simulink model "lab4_4"  (R2017b)
settings: Solver=VariableStepAuto  StartTime=0.0  StopTime=4  RelTol=1e-3
settings Model: Creator=yoel_  LastModifiedBy=yoel_

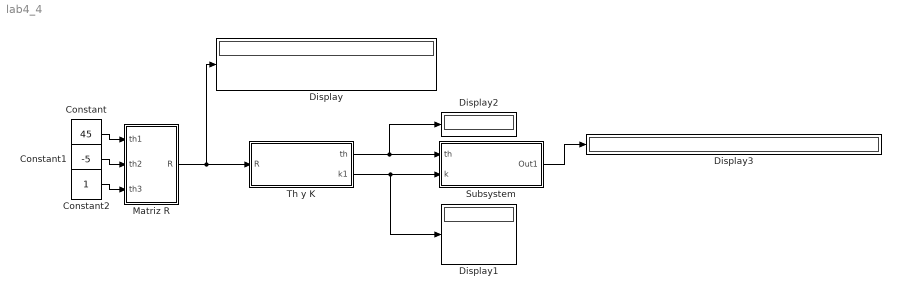
== system lab4_4 ==
  Constant : Constant  Value=45
  Constant1 : Constant  Value=-5
  Constant2 : Constant
  Display{,1..3} (4 alike) : Display
  Matriz R : Subsystem
  Subsystem : Subsystem
  Th y K : Subsystem
  wires:
  Constant/1 -> Matriz R/1(th1)
  Constant1/1 -> Matriz R/2(th2)
  Constant2/1 -> Matriz R/3(th3)
  Matriz R/1(R) -> Th y K/1("R "), Display/1
  Th y K/2(k1) -> Subsystem/2("k "), Display1/1
  Th y K/1("th ") -> Subsystem/1("th "), Display2/1
  Subsystem/1(Out1) -> Display3/1

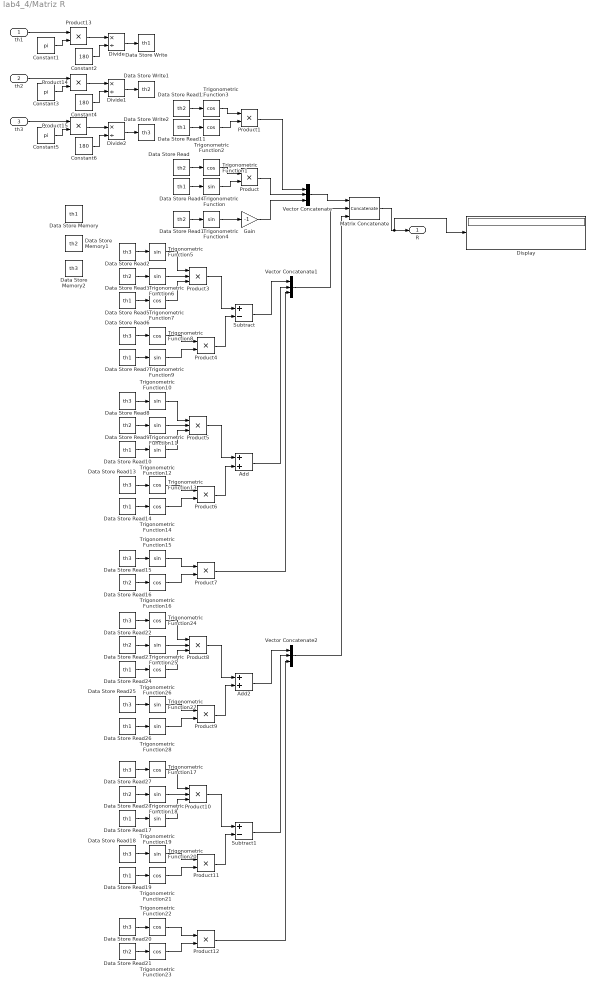
== system lab4_4/Matriz R ==
  th1 : Inport
  th2 : Inport  Port=2
  th3 : Inport  Port=3
  Add : Sum
  Add2 : Sum
  Constant1 : Constant  Value=pi
  Constant2 : Constant  Value=180
  Constant3 : Constant  Value=pi
  Constant4 : Constant  Value=180
  Constant5 : Constant  Value=pi
  Constant6 : Constant  Value=180
  Data Store Memory : DataStoreMemory  DataStoreName=th1  ReadBeforeWriteMsg=warning  WriteAfterWriteMsg=warning  WriteAfterReadMsg=warning  ShowAdditionalParam=off
  Data Store Memory1 : DataStoreMemory  DataStoreName=th2  ReadBeforeWriteMsg=warning  WriteAfterWriteMsg=warning  WriteAfterReadMsg=warning  ShowAdditionalParam=off
  Data Store Memory2 : DataStoreMemory  DataStoreName=th3  ReadBeforeWriteMsg=warning  WriteAfterWriteMsg=warning  WriteAfterReadMsg=warning  ShowAdditionalParam=off
  Data Store Read{,1,3,9,12,16,21,23,28} (9 alike) : DataStoreRead  DataStoreName=th2
  Data Store Read{4..5,7,10..11,14,17,19,24,26} (10 alike) : DataStoreRead  DataStoreName=th1
  Data Store Read{2,6,8,13,15,18,20,22,25,27} (10 alike) : DataStoreRead  DataStoreName=th3
  Data Store Write : DataStoreWrite  DataStoreName=th1
  Data Store Write1 : DataStoreWrite  DataStoreName=th2
  Data Store Write2 : DataStoreWrite  DataStoreName=th3
  Display : Display
  Divide : Product  Inputs=*/
  Divide1 : Product  Inputs=*/
  Divide2 : Product  Inputs=*/
  Gain : Gain  Gain=-1
  Matrix Concatenate : Concatenate  NumInputs=3  ConcatenateDimension=3
  Product{,1,4,6..7,9,11..15} (11 alike) : Product
  Product{3,5,8,10} (4 alike) : Product  Inputs=3
  Subtract : Sum  Inputs=+-
  Subtract1 : Sum  Inputs=+-
  Trigonometric Function{,4..6,9..12,15,18..20,25,27..28} (15 alike) : Trigonometry
  Trigonometric Function{1..3,7..8,13..14,16..17,21..24,26} (14 alike) : Trigonometry  Operator=cos
  Vector Concatenate : Concatenate  NumInputs=3
  Vector Concatenate1 : Concatenate  NumInputs=3
  Vector Concatenate2 : Concatenate  NumInputs=3
  R : Outport
  wires:
  Trigonometric Function3/1 -> Product1/1
  Trigonometric Function/1 -> Product/2
  Trigonometric Function2/1 -> Product1/2
  Trigonometric Function1/1 -> Product/1
  Trigonometric Function4/1 -> Gain/1
  Data Store Read12/1 -> Trigonometric Function3/1
  Data Store Read11/1 -> Trigonometric Function2/1
  Data Store Read/1 -> Trigonometric Function1/1
  Data Store Read4/1 -> Trigonometric Function/1
  Data Store Read1/1 -> Trigonometric Function4/1
  Product1/1 -> Vector Concatenate/1
  Product/1 -> Vector Concatenate/2
  Gain/1 -> Vector Concatenate/3
  Vector Concatenate/1 -> Matrix Concatenate/1
  Vector Concatenate1/1 -> Matrix Concatenate/2
  Matrix Concatenate/1 -> Display/1, R/1
  Data Store Read2/1 -> Trigonometric Function5/1
  Data Store Read3/1 -> Trigonometric Function6/1
  Data Store Read5/1 -> Trigonometric Function7/1
  Trigonometric Function5/1 -> Product3/1
  Trigonometric Function6/1 -> Product3/2
  Trigonometric Function7/1 -> Product3/3
  Product3/1 -> Subtract/1
  Data Store Read6/1 -> Trigonometric Function8/1
  Data Store Read7/1 -> Trigonometric Function9/1
  Trigonometric Function8/1 -> Product4/1
  Trigonometric Function9/1 -> Product4/2
  Product4/1 -> Subtract/2
  Subtract/1 -> Vector Concatenate1/1
  Product6/1 -> Add/2
  Trigonometric Function11/1 -> Product5/2
  Data Store Read9/1 -> Trigonometric Function11/1
  Trigonometric Function14/1 -> Product6/2
  Trigonometric Function12/1 -> Product5/3
  Data Store Read14/1 -> Trigonometric Function14/1
  Data Store Read10/1 -> Trigonometric Function12/1
  Trigonometric Function13/1 -> Product6/1
  Product5/1 -> Add/1
  Data Store Read8/1 -> Trigonometric Function10/1
  Trigonometric Function10/1 -> Product5/1
  Data Store Read13/1 -> Trigonometric Function13/1
  Add/1 -> Vector Concatenate1/2
  Data Store Read15/1 -> Trigonometric Function15/1
  Data Store Read16/1 -> Trigonometric Function16/1
  Trigonometric Function15/1 -> Product7/1
  Trigonometric Function16/1 -> Product7/2
  Product7/1 -> Vector Concatenate1/3
  Product12/1 -> Vector Concatenate2/3
  Trigonometric Function23/1 -> Product12/2
  Trigonometric Function22/1 -> Product12/1
  Data Store Read21/1 -> Trigonometric Function23/1
  Data Store Read20/1 -> Trigonometric Function22/1
  Subtract1/1 -> Vector Concatenate2/2
  Data Store Read18/1 -> Trigonometric Function20/1
  Trigonometric Function17/1 -> Product10/1
  Data Store Read27/1 -> Trigonometric Function17/1
  Product10/1 -> Subtract1/1
  Trigonometric Function20/1 -> Product11/1
  Data Store Read17/1 -> Trigonometric Function19/1
  Data Store Read19/1 -> Trigonometric Function21/1
  Trigonometric Function19/1 -> Product10/3
  Trigonometric Function21/1 -> Product11/2
  Data Store Read28/1 -> Trigonometric Function18/1
  Trigonometric Function18/1 -> Product10/2
  Product11/1 -> Subtract1/2
  Add2/1 -> Vector Concatenate2/1
  Product9/1 -> Add2/2
  Trigonometric Function28/1 -> Product9/2
  Trigonometric Function27/1 -> Product9/1
  Data Store Read26/1 -> Trigonometric Function28/1
  Data Store Read25/1 -> Trigonometric Function27/1
  Product8/1 -> Add2/1
  Trigonometric Function26/1 -> Product8/3
  Trigonometric Function25/1 -> Product8/2
  Trigonometric Function24/1 -> Product8/1
  Data Store Read24/1 -> Trigonometric Function26/1
  Data Store Read23/1 -> Trigonometric Function25/1
  Data Store Read22/1 -> Trigonometric Function24/1
  Vector Concatenate2/1 -> Matrix Concatenate/3
  th1/1 -> Product13/1
  Constant1/1 -> Product13/2
  Product13/1 -> Divide/1
  Constant2/1 -> Divide/2
  Divide/1 -> Data Store Write/1
  Divide1/1 -> Data Store Write1/1
  Constant4/1 -> Divide1/2
  Product14/1 -> Divide1/1
  Constant3/1 -> Product14/2
  th2/1 -> Product14/1
  th3/1 -> Product15/1
  Constant5/1 -> Product15/2
  Product15/1 -> Divide2/1
  Constant6/1 -> Divide2/2
  Divide2/1 -> Data Store Write2/1

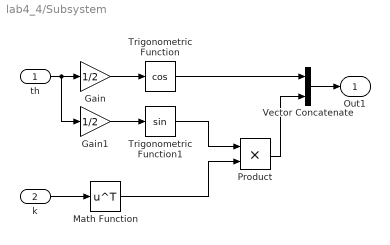
== system lab4_4/Subsystem ==
  "th " : Inport
  "k " : Inport  Port=2
  Gain : Gain  Gain=1/2
  Gain1 : Gain  Gain=1/2
  Math Function : Math  Operator=transpose  SaturateOnIntegerOverflow=on
  Product : Product
  Trigonometric Function : Trigonometry  Operator=cos
  Trigonometric Function1 : Trigonometry
  Vector Concatenate : Concatenate
  Out1 : Outport
  wires:
  "th "/1 -> Gain1/1, Gain/1
  Gain/1 -> Trigonometric Function/1
  Gain1/1 -> Trigonometric Function1/1
  "k "/1 -> Math Function/1
  Trigonometric Function1/1 -> Product/1
  Math Function/1 -> Product/2
  Product/1 -> Vector Concatenate/2
  Trigonometric Function/1 -> Vector Concatenate/1
  Vector Concatenate/1 -> Out1/1

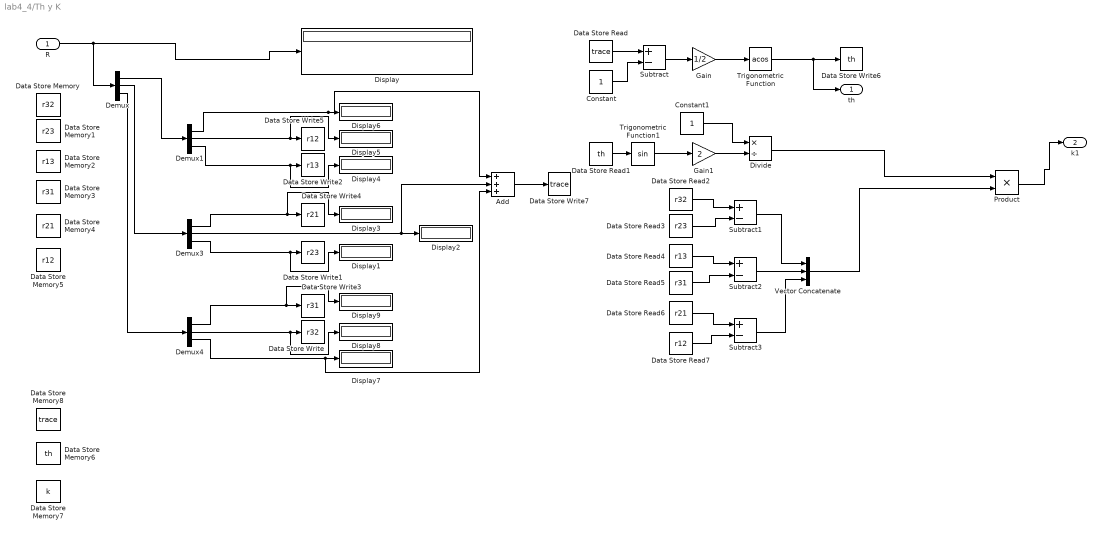
== system lab4_4/Th y K ==
  "R " : Inport
  Add : Sum  Inputs=3
  Constant : Constant
  Constant1 : Constant
  Data Store Memory : DataStoreMemory  DataStoreName=r32  ReadBeforeWriteMsg=warning  WriteAfterWriteMsg=warning  WriteAfterReadMsg=warning  ShowAdditionalParam=off
  Data Store Memory1 : DataStoreMemory  DataStoreName=r23  ReadBeforeWriteMsg=warning  WriteAfterWriteMsg=warning  WriteAfterReadMsg=warning  ShowAdditionalParam=off
  Data Store Memory2 : DataStoreMemory  DataStoreName=r13  ReadBeforeWriteMsg=warning  WriteAfterWriteMsg=warning  WriteAfterReadMsg=warning  ShowAdditionalParam=off
  Data Store Memory3 : DataStoreMemory  DataStoreName=r31  ReadBeforeWriteMsg=warning  WriteAfterWriteMsg=warning  WriteAfterReadMsg=warning  ShowAdditionalParam=off
  Data Store Memory4 : DataStoreMemory  DataStoreName=r21  ReadBeforeWriteMsg=warning  WriteAfterWriteMsg=warning  WriteAfterReadMsg=warning  ShowAdditionalParam=off
  Data Store Memory5 : DataStoreMemory  DataStoreName=r12  ReadBeforeWriteMsg=warning  WriteAfterWriteMsg=warning  WriteAfterReadMsg=warning  ShowAdditionalParam=off
  Data Store Memory6 : DataStoreMemory  DataStoreName=th  ReadBeforeWriteMsg=warning  WriteAfterWriteMsg=warning  WriteAfterReadMsg=warning  ShowAdditionalParam=off
  Data Store Memory7 : DataStoreMemory  DataStoreName=k  ReadBeforeWriteMsg=warning  WriteAfterWriteMsg=warning  WriteAfterReadMsg=warning  ShowAdditionalParam=off
  Data Store Memory8 : DataStoreMemory  DataStoreName=trace  ReadBeforeWriteMsg=warning  WriteAfterWriteMsg=warning  WriteAfterReadMsg=warning  ShowAdditionalParam=off
  Data Store Read : DataStoreRead  DataStoreName=trace
  Data Store Read1 : DataStoreRead  DataStoreName=th
  Data Store Read2 : DataStoreRead  DataStoreName=r32
  Data Store Read3 : DataStoreRead  DataStoreName=r23
  Data Store Read4 : DataStoreRead  DataStoreName=r13
  Data Store Read5 : DataStoreRead  DataStoreName=r31
  Data Store Read6 : DataStoreRead  DataStoreName=r21
  Data Store Read7 : DataStoreRead  DataStoreName=r12
  Data Store Write : DataStoreWrite  DataStoreName=r32
  Data Store Write1 : DataStoreWrite  DataStoreName=r23
  Data Store Write2 : DataStoreWrite  DataStoreName=r13
  Data Store Write3 : DataStoreWrite  DataStoreName=r31
  Data Store Write4 : DataStoreWrite  DataStoreName=r21
  Data Store Write5 : DataStoreWrite  DataStoreName=r12
  Data Store Write6 : DataStoreWrite  DataStoreName=th
  Data Store Write7 : DataStoreWrite  DataStoreName=trace
  Demux{,1,3..4} (4 alike) : Demux  Outputs=3
  Display{,1..9} (10 alike) : Display
  Divide : Product  Inputs=*/
  Gain : Gain  Gain=1/2
  Gain1 : Gain  Gain=2
  Product : Product
  Subtract{,1..3} (4 alike) : Sum  Inputs=+-
  Trigonometric Function : Trigonometry  Operator=acos
  Trigonometric Function1 : Trigonometry
  Vector Concatenate : Concatenate  NumInputs=3  Mode=Multidimensional array
  "th " : Outport
  k1 : Outport  Port=2
  wires:
  "R "/1 -> Demux/1, Display/1
  Demux/2 -> Demux3/1
  Demux/3 -> Demux4/1
  Demux/1 -> Demux1/1
  Demux1/3 -> Data Store Write2/1, Display4/1
  Demux1/1 -> Add/1, Display6/1
  Demux3/2 -> Display2/1, Add/2
  Demux3/1 -> Data Store Write4/1, Display3/1
  Demux3/3 -> Display1/1, Data Store Write1/1
  Demux4/1 -> Data Store Write3/1, Display9/1
  Demux4/3 -> Add/3, Display7/1
  Demux4/2 -> Display8/1, Data Store Write/1
  Demux1/2 -> Data Store Write5/1, Display5/1
  Add/1 -> Data Store Write7/1
  Data Store Read/1 -> Subtract/1
  Constant/1 -> Subtract/2
  Subtract/1 -> Gain/1
  Gain/1 -> Trigonometric Function/1
  Trigonometric Function/1 -> "th "/1, Data Store Write6/1
  Trigonometric Function1/1 -> Gain1/1
  Data Store Read1/1 -> Trigonometric Function1/1
  Gain1/1 -> Divide/2
  Constant1/1 -> Divide/1
  Data Store Read2/1 -> Subtract1/1
  Data Store Read3/1 -> Subtract1/2
  Data Store Read4/1 -> Subtract2/1
  Data Store Read5/1 -> Subtract2/2
  Data Store Read7/1 -> Subtract3/2
  Data Store Read6/1 -> Subtract3/1
  Vector Concatenate/1 -> Product/2
  Subtract1/1 -> Vector Concatenate/1
  Subtract3/1 -> Vector Concatenate/3
  Subtract2/1 -> Vector Concatenate/2
  Divide/1 -> Product/1
  Product/1 -> k1/1
